simulink model "PIDF_avec_xy_pour_algo2"  (R2023a)
settings: Solver=VariableStepAuto  StartTime=0.0  StopTime=100  RelTol=1e-3
values from neighbouring files (symbols this model uses):
  Ca2 = [1 0 0 0 0 0 0 0 0 0 0 0; 0 1 0 0 0 0 0 0 0 0 0 0; 0 0 1 0 0 0 0 0 0 0 0 0; 0 0 0 0 0 0 1 0 0 0 0 0; 0 0 0 0 0 0 0 1 0 0 0 0; 0 0 0 0 0 0 0 0 1 0 0 0]    [constants.m]
  Ccp2 = [0 0 0 1 0 0; 0 0 0 0 1 0]    [constants.m]
  g = 9.81    [constants.m]
  k = 3.1582e-10    [constants.m]
  m = 28.6e-3    (= 0.0286)    [constants.m]
  M = [1 1 1 1 ; 0 -1 0 1 ; 1 0 -1 0 ; -1 1 -1 1]    [constants.m]
libraries: cstblocks x6
settings Model: Creator=raphb  LastModifiedBy=raphb

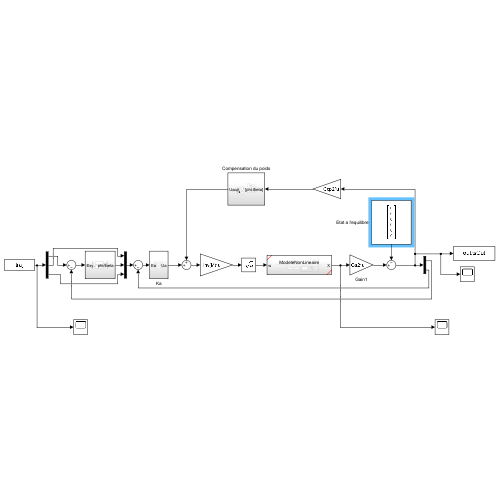
[thumbnail: Simulink's stored preview of the top-level diagram]
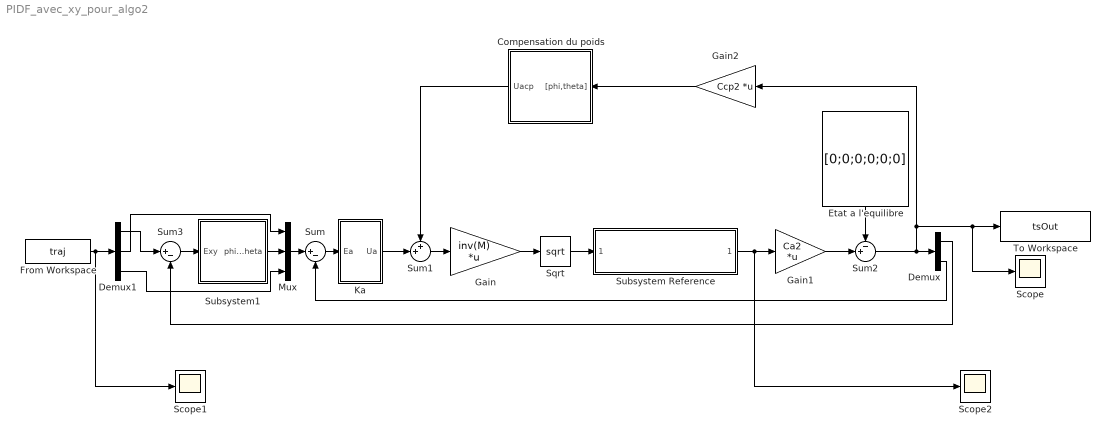
== system PIDF_avec_xy_pour_algo2 ==
  Compensation du poids : Subsystem
  Demux : Demux  Outputs=[2;4]
  Demux1 : Demux  Outputs=[2;1;1]
  Etat a l'equilibre : Constant  Value=[0;0;0;0;0;0]  VectorParams1D=off
  From Workspace : FromWorkspace  VariableName=traj
  Gain : Gain  Gain=inv(M)  Multiplication=Matrix(K*u)
  Gain1 : Gain  Gain=Ca2  Multiplication=Matrix(K*u)
  Gain2 : Gain  Gain=Ccp2  Multiplication=Matrix(K*u)
  Ka : Subsystem
  Mux : Mux  Inputs=[1;2;1]
  Scope : Scope
  Scope1 : Scope
  Scope2 : Scope
  Sqrt : Sqrt
  Subsystem Reference : Subsystem  ReferencedSubsystem=ModeleNonLineaire
  Subsystem1 : Subsystem
  Sum : Sum  Inputs=|+-
  Sum1 : Sum  Inputs=++|
  Sum2 : Sum  Inputs=-+|
  Sum3 : Sum  Inputs=|+-
  To Workspace : ToWorkspace  VariableName=tsOut  SaveFormat=Timeseries  SampleTime=-1
  wires:
  Compensation du poids/1(Uacp) -> Sum1/1
  Etat a l'equilibre/1 -> Sum2/1
  Gain/1 -> Sqrt/1
  Gain1/1 -> Sum2/2
  Subsystem Reference/1 -> Scope2/1, Gain1/1
  Sum2/1 -> Gain2/1, Scope/1, To Workspace/1, Demux/1
  Sum1/1 -> Gain/1
  Ka/1(Ua) -> Sum1/2
  Sqrt/1 -> Subsystem Reference/1
  Sum/1 -> Ka/1(Ea)
  Gain2/1 -> Compensation du poids/1("[phi,theta]")
  Demux/2 -> Sum/2
  Demux/1 -> Sum3/2
  Demux1/1 -> Sum3/1
  Sum3/1 -> Subsystem1/1(Exy)
  Subsystem1/1(phi/theta) -> Mux/2
  Mux/1 -> Sum/1
  Demux1/2 -> Mux/1
  Demux1/3 -> Mux/3
  From Workspace/1 -> Scope1/1, Demux1/1

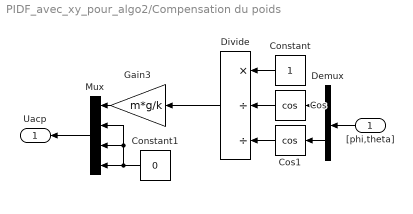
== system PIDF_avec_xy_pour_algo2/Compensation du poids ==
  "[phi,theta]" : Inport
  Constant : Constant
  Constant1 : Constant  Value=0
  Cos : Trigonometry  Operator=cos
  Cos1 : Trigonometry  Operator=cos
  Demux : Demux  Outputs=2
  Divide : Product  Inputs=*//
  Gain3 : Gain  Gain=m*g/k
  Mux : Mux
  Uacp : Outport
  wires:
  Cos1/1 -> Divide/3
  Cos/1 -> Divide/2
  Demux/1 -> Cos/1
  "[phi,theta]"/1 -> Demux/1
  Demux/2 -> Cos1/1
  Constant/1 -> Divide/1
  Gain3/1 -> Mux/1
  Mux/1 -> Uacp/1
  Constant1/1 -> Mux/2, Mux/3, Mux/4
  Divide/1 -> Gain3/1

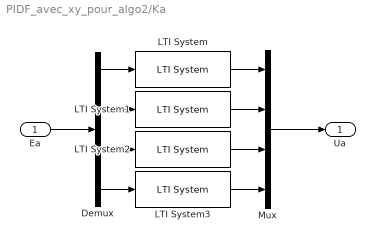
== system PIDF_avec_xy_pour_algo2/Ka ==
  Ea : Inport
  Demux : Demux
  LTI System : cstblocks/LTI System  sys=Kz  IC=[]
  LTI System1 : cstblocks/LTI System  sys=Kphi  IC=[]
  LTI System2 : cstblocks/LTI System  sys=Ktheta  IC=[]
  LTI System3 : cstblocks/LTI System  sys=Kpsi  IC=[]
  Mux : Mux
  Ua : Outport
  wires:
  LTI System1/1 -> Mux/2
  Demux/4 -> LTI System3/1
  Demux/3 -> LTI System2/1
  LTI System/1 -> Mux/1
  LTI System3/1 -> Mux/4
  Ea/1 -> Demux/1
  Demux/2 -> LTI System1/1
  LTI System2/1 -> Mux/3
  Demux/1 -> LTI System/1
  Mux/1 -> Ua/1

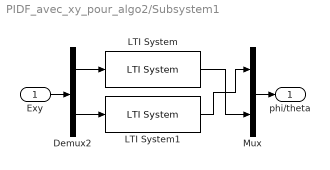
== system PIDF_avec_xy_pour_algo2/Subsystem1 ==
  Exy : Inport
  Demux2 : Demux  Outputs=2
  LTI System : cstblocks/LTI System  sys=Kx  IC=[]
  LTI System1 : cstblocks/LTI System  sys=Ky  IC=[]
  Mux : Mux  Inputs=2
  phi/theta : Outport
  wires:
  LTI System/1 -> Mux/2
  LTI System1/1 -> Mux/1
  Demux2/1 -> LTI System/1
  Exy/1 -> Demux2/1
  Demux2/2 -> LTI System1/1
  Mux/1 -> phi/theta/1
